simulink model "doble_pendulo"  (R2023a)
settings: Solver=VariableStepAuto  StartTime=0  StopTime=10.0  MaxStep=0.01  RelTol=1e-3
values from neighbouring files (symbols this model uses):
  g = 9.81    [Practica_1_doble_pendulo.m]
  l1 = 0.3    [Practica_1_doble_pendulo.m]
  l2 = 0.25    [Practica_1_doble_pendulo.m]
  m1 = 0.2    [Practica_1_doble_pendulo.m]
  m2 = 0.1    [Practica_1_doble_pendulo.m]
settings Model: Creator=penqu  LastModifiedBy=penqu

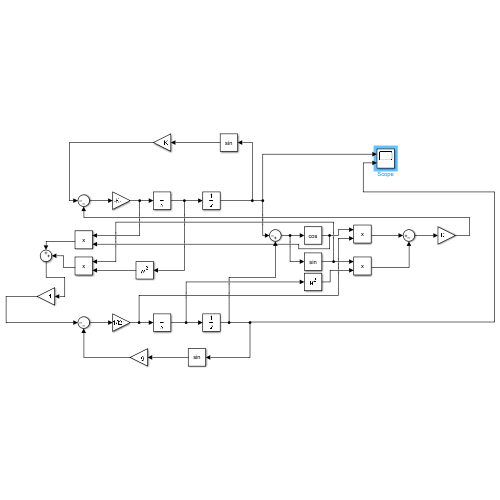
[thumbnail: Simulink's stored preview of the top-level diagram]
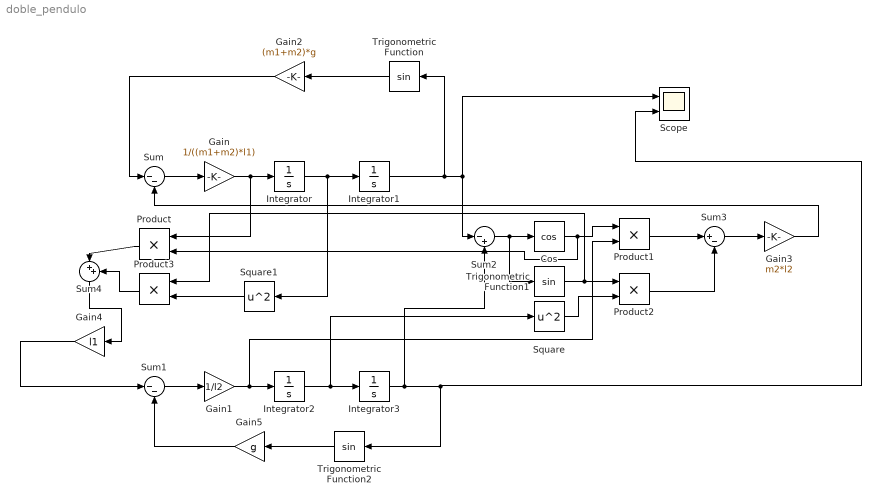
== system doble_pendulo ==
  Cos : Trigonometry  Operator=cos
  Gain : Gain  Gain=1/((m1+m2)*l1)
  Gain1 : Gain  Gain=1/l2
  Gain2 : Gain  Gain=(m1+m2)*g
  Gain3 : Gain  Gain=m2*l2
  Gain4 : Gain  Gain=l1
  Gain5 : Gain  Gain=g
  Integrator : Integrator
  Integrator1 : Integrator
  Integrator2 : Integrator
  Integrator3 : Integrator  InitialCondition=(35*pi)/180
  Product{,1..3} (4 alike) : Product
  Scope : Scope  NumInputPorts=2
  Square : Math  Operator=square
  Square1 : Math  Operator=square
  Sum : Sum  Inputs=|--
  Sum1 : Sum  Inputs=|--
  Sum2 : Sum  Inputs=|-+
  Sum3 : Sum  Inputs=|+-
  Sum4 : Sum  Inputs=|++
  Trigonometric Function : Trigonometry
  Trigonometric Function1 : Trigonometry
  Trigonometric Function2 : Trigonometry
  wires:
  Sum/1 -> Gain/1
  Gain/1 -> Product/1, Integrator/1
  Integrator/1 -> Square1/1, Integrator1/1
  Integrator1/1 -> Trigonometric Function/1, Sum2/1, Scope/1
  Sum1/1 -> Gain1/1
  Gain1/1 -> Product1/2, Integrator2/1
  Integrator2/1 -> Square/1, Integrator3/1
  Trigonometric Function/1 -> Gain2/1
  Gain2/1 -> Sum/1
  Sum2/1 -> Trigonometric Function1/1, Cos/1
  Cos/1 -> Product/2, Product1/1
  Product1/1 -> Sum3/1
  Trigonometric Function1/1 -> Product3/1, Product2/1
  Square/1 -> Product2/2
  Product2/1 -> Sum3/2
  Sum3/1 -> Gain3/1
  Gain3/1 -> Sum/2
  Square1/1 -> Product3/2
  Sum4/1 -> Gain4/1
  Gain4/1 -> Sum1/1
  Trigonometric Function2/1 -> Gain5/1
  Gain5/1 -> Sum1/2
  Integrator3/1 -> Sum2/2, Scope/2, Trigonometric Function2/1
  Product/1 -> Sum4/1
  Product3/1 -> Sum4/2
